simulink model "QUAD_EULER_MPC_FTSMC3"  (R2024b)
settings: Solver=ode1  StartTime=0.0  StopTime=30  FixedStep=0.001  RelTol=1e-3
values from neighbouring files (symbols this model uses):
  F1 = F1 + 2*(PSI_I'*C'*Q_z*C*PHI_I)    [Setup_MPC_SMC_Drone.m]
  F1_xy = F1_xy + 2*(PSI_xy_I'*C_xy'*Q_xy*C_xy*PHI_xy_I)    [Setup_MPC_SMC_Drone.m]
  F2 = F2 - 2*(PSI_I'*C'*Q_z*pi_n)    [Setup_MPC_SMC_Drone.m]
  F2_xy = F2_xy - 2*(PSI_xy_I'*C_xy'*Q_xy*pi_n)    [Setup_MPC_SMC_Drone.m]
  F3 = F3 - 2*(pi_nu'*Qt_z)    [Setup_MPC_SMC_Drone.m]
  F3_xy = F3_xy - 2*(pi_nu'*R_xy)    [Setup_MPC_SMC_Drone.m]
  F4 = F4 + 2*(PSI_I'*C'*Qt_z*C*SumG)    [Setup_MPC_SMC_Drone.m]
  g = 9.81    [Setup_MPC_SMC_Drone.m]
  G = [0;-g]    [Setup_MPC_SMC_Drone.m]
  H = H + 2*(PSI_I'*C'*Q_z*C*PSI_I + pi_nu'*Qt_z*pi_nu)    [Setup_MPC_SMC_Drone.m]
  H_xy = H_xy + 2*(PSI_xy_I'*C_xy'*Q_xy*C_xy*PSI_xy_I + pi_nu'*R_xy*pi_nu)    [Setup_MPC_SMC_Drone.m]
  J = diag([Jxx Jyy Jzz])    [Setup_MPC_SMC_Drone.m]
  m = 1.121    [Setup_MPC_SMC_Drone.m]
  N = 10    [Setup_MPC_SMC_Drone.m]
  N_xy = 10    [Setup_MPC_SMC_Drone.m]
  ny = size(C,1)    [Setup_MPC_SMC_Drone.m]
  ny_xy = size(C_xy,1)    [Setup_MPC_SMC_Drone.m]
  u_des = 0    [Setup_MPC_SMC_Drone.m]
  u_des_xy = [0;0]    [Setup_MPC_SMC_Drone.m]
undefined symbols (not defined in the file or in its folder): A_l, B_l, C_l, N_l, nr_l, nu, nu_l, phi_l, psi_l, Qu_l, Qy_l, ud_l
libraries: matrix_library x2, aerolibutil x2
settings Model: Creator=Jorge  LastModifiedBy=dr.gerardocastanon

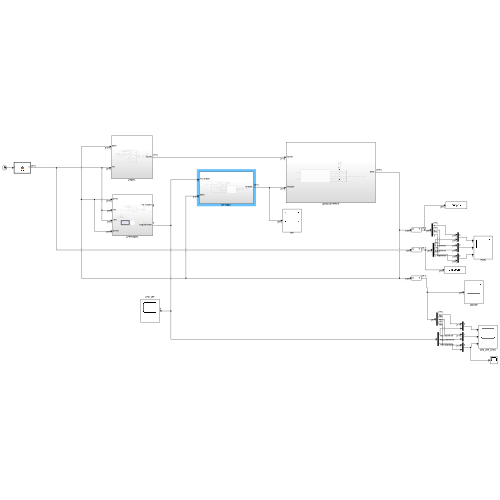
[thumbnail: Simulink's stored preview of the top-level diagram]
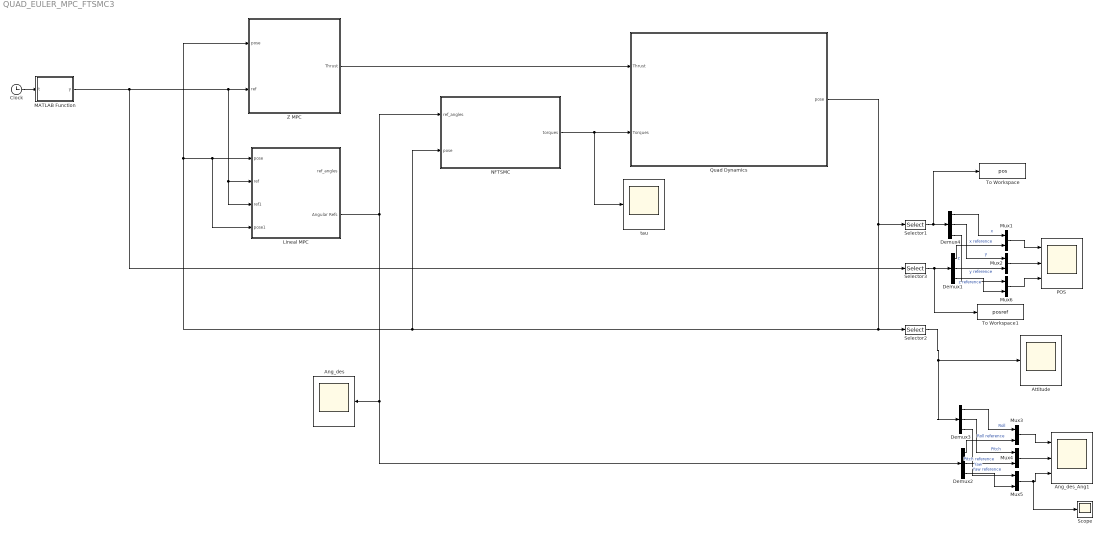
== system QUAD_EULER_MPC_FTSMC3 ==
  Ang_des : Scope
  Ang_des_Ang1 : Scope  NumInputPorts=3
  Attitude : Scope
  Clock : Clock
  Demux{1..4} (4 alike) : Demux  Outputs=3
  Lineal MPC : Subsystem
  MATLAB Function : MATLAB Function  TreatAsAtomicUnit=on
  Mux{1..6} (6 alike) : Mux  Inputs=2
  NFTSMC : Subsystem
  POS : Scope  NumInputPorts=3
  Quad Dynamics : Subsystem
  Scope : Scope
  Selector1 : Selector  InputPortWidth=15  IndexOptions=Starting index (dialog)  Indices=[1]  OutputSizes=3
  Selector2 : Selector  InputPortWidth=15  IndexOptions=Starting index (dialog)  Indices=[10]  OutputSizes=3
  Selector3 : Selector  InputPortWidth=4  IndexOptions=Starting index (dialog)  Indices=[1]  OutputSizes=3
  To Workspace : ToWorkspace  VariableName=pos  SampleTime=-1
  To Workspace1 : ToWorkspace  VariableName=posref  SampleTime=-1
  Z MPC : Subsystem
  tau : Scope
  wires:
  Quad Dynamics/1(pose) -> Selector1/1, Selector2/1, NFTSMC/2(pose), Z MPC/1(pose), Lineal MPC/4(pose1), Lineal MPC/1(pose)
  Z MPC/1(Thrust) -> Quad Dynamics/1(Thrust)
  MATLAB Function/1(y) -> Z MPC/2(ref), Lineal MPC/3(ref1), Lineal MPC/2(ref), Selector3/1
  Clock/1 -> MATLAB Function/1(t)
  Mux4/1 -> Ang_des_Ang1/2
  Mux5/1 -> Scope/1, Ang_des_Ang1/3
  Mux3/1 -> Ang_des_Ang1/1
  Mux2/1 -> POS/2
  Mux6/1 -> POS/3
  Mux1/1 -> POS/1
  Selector1/1 -> To Workspace/1, Demux4/1
  Selector3/1 -> To Workspace1/1, Demux1/1
  Demux3/1 -> Mux3/1  "Roll"
  Demux3/2 -> Mux4/1  "Pitch"
  Demux2/1 -> Mux3/2  "Roll reference"
  Demux3/3 -> Mux5/1  "Yaw"
  Demux2/2 -> Mux4/2  "Pitch reference"
  Demux2/3 -> Mux5/2  "Yaw reference"
  Demux4/1 -> Mux1/1  "x"
  Demux4/2 -> Mux2/1  "y"
  Demux1/1 -> Mux1/2  "x reference"
  Demux4/3 -> Mux6/1  "z"
  Demux1/2 -> Mux2/2  "y reference"
  Demux1/3 -> Mux6/2  "z reference"
  NFTSMC/1(torques) -> tau/1, Quad Dynamics/2(Torques)
  Selector2/1 -> Demux3/1, Attitude/1
  Lineal MPC/2(Angular Refs) -> Demux2/1, Ang_des/1, NFTSMC/1(ref_angles)

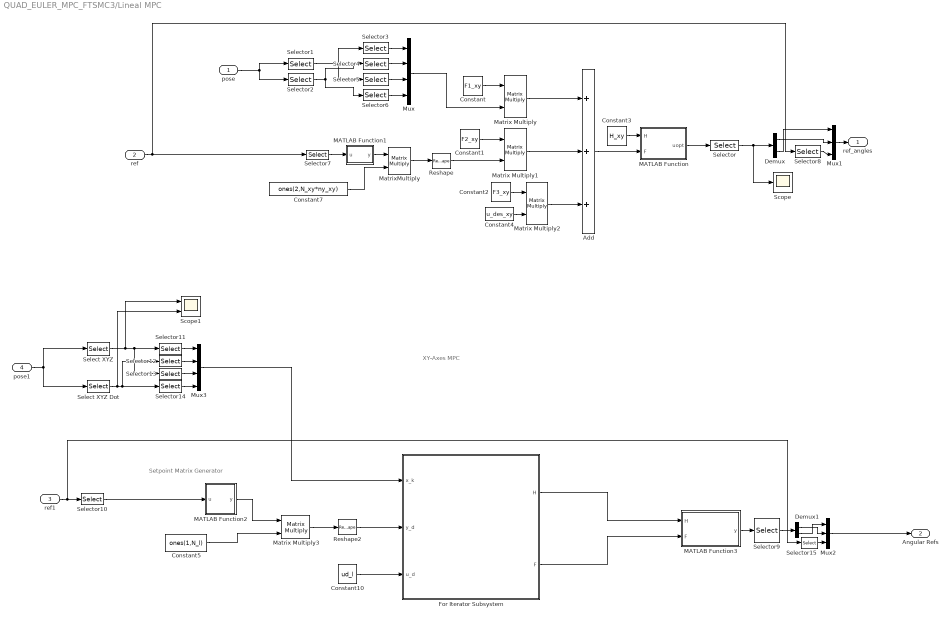
== system QUAD_EULER_MPC_FTSMC3/Lineal MPC ==
  note: Setpoint Matrix Generator
  note: XY-Axes MPC
  pose : Inport
  ref : Inport  Port=2
  ref1 : Inport  Port=3
  pose1 : Inport  Port=4
  Add : Sum  Inputs=+++
  Constant : Constant  Value=F1_xy
  Constant1 : Constant  Value=F2_xy
  Constant10 : Constant  Value=ud_l  VectorParams1D=off
  Constant2 : Constant  Value=F3_xy
  Constant3 : Constant  Value=H_xy
  Constant4 : Constant  Value=u_des_xy
  Constant5 : Constant  Value=ones(1,N_l)  VectorParams1D=off
  Constant7 : Constant  Value=ones(2,N_xy*ny_xy)
  Demux : Demux  Outputs=2
  Demux1 : Demux  Outputs=2
  For Iterator Subsystem : Subsystem  TreatAsAtomicUnit=on
  MATLAB Function : MATLAB Function  TreatAsAtomicUnit=on
  MATLAB Function1 : MATLAB Function  TreatAsAtomicUnit=on
  MATLAB Function2 : MATLAB Function  TreatAsAtomicUnit=on
  MATLAB Function3 : MATLAB Function  TreatAsAtomicUnit=on
  Matrix Multiply{,1..3} (4 alike) : Product  Multiplication=Matrix(*)
  MatrixMultiply : Product  Multiplication=Matrix(*)
  Mux : Mux
  Mux1 : Mux  Inputs=3
  Mux2 : Mux  Inputs=3
  Mux3 : Mux
  Reshape : Reshape  OutputDimensionality=Customize  OutputDimensions=[N_xy*ny_xy,1]
  Reshape2 : Reshape  OutputDimensionality=Customize  OutputDimensions=[N_l*nr_l,1]
  Scope : Scope
  Scope1 : Scope  NumInputPorts=2
  Select XYZ : Selector  InputPortWidth=15  IndexOptions=Index vector (dialog)  Indices=[1:3]  OutputSizes=1
  Select XYZ Dot : Selector  InputPortWidth=15  IndexOptions=Index vector (dialog)  Indices=[4:6]  OutputSizes=1
  Selector : Selector  InputPortWidth=20  IndexOptions=Starting index (dialog)  Indices=1  OutputSizes=2
  Selector1 : Selector  InputPortWidth=15  IndexOptions=Index vector (dialog)  Indices=[1 2]  OutputSizes=1
  Selector10 : Selector  InputPortWidth=4  IndexOptions=Index vector (dialog)  Indices=[1:2]  OutputSizes=1
  Selector11 : Selector  InputPortWidth=3  IndexOptions=Index vector (dialog)  Indices=[1]  OutputSizes=1
  Selector12 : Selector  InputPortWidth=3  IndexOptions=Index vector (dialog)  Indices=[1]  OutputSizes=1
  Selector13 : Selector  InputPortWidth=3  IndexOptions=Index vector (dialog)  Indices=[2]  OutputSizes=1
  Selector14 : Selector  InputPortWidth=3  IndexOptions=Index vector (dialog)  Indices=[2]  OutputSizes=1
  Selector15 : Selector  InputPortWidth=4  IndexOptions=Index vector (dialog)  Indices=4  OutputSizes=1
  Selector2 : Selector  InputPortWidth=15  IndexOptions=Index vector (dialog)  Indices=[4 5]  OutputSizes=1
  Selector3 : Selector  InputPortWidth=2  IndexOptions=Index vector (dialog)  Indices=1  OutputSizes=1
  Selector4 : Selector  InputPortWidth=2  IndexOptions=Index vector (dialog)  Indices=1  OutputSizes=1
  Selector5 : Selector  InputPortWidth=2  IndexOptions=Index vector (dialog)  Indices=2  OutputSizes=1
  Selector6 : Selector  InputPortWidth=2  IndexOptions=Index vector (dialog)  Indices=1  OutputSizes=1
  Selector7 : Selector  InputPortWidth=4  IndexOptions=Index vector (dialog)  Indices=[1:2]  OutputSizes=1
  Selector8 : Selector  InputPortWidth=4  IndexOptions=Index vector (dialog)  Indices=4  OutputSizes=1
  Selector9 : Selector  InputPortWidth=N_l*nu_l  IndexOptions=Index vector (dialog)  Indices=[1:2]  OutputSizes=1
  ref_angles : Outport
  Angular Refs : Outport  Port=2
  wires:
  Constant3/1 -> MATLAB Function/1(H)
  Add/1 -> MATLAB Function/2(F)
  MATLAB Function/1(uopt) -> Selector/1
  Selector/1 -> Demux/1, Scope/1
  pose/1 -> Selector2/1, Selector1/1
  Selector1/1 -> Selector3/1, Selector5/1
  Selector2/1 -> Selector4/1, Selector6/1
  Selector3/1 -> Mux/1
  Selector4/1 -> Mux/2
  Selector5/1 -> Mux/3
  Selector6/1 -> Mux/4
  Constant/1 -> Matrix Multiply/1
  Mux/1 -> Matrix Multiply/2
  Matrix Multiply/1 -> Add/1
  Matrix Multiply1/1 -> Add/2
  Constant1/1 -> Matrix Multiply1/1
  Constant7/1 -> MatrixMultiply/2
  ref/1 -> Selector8/1, Selector7/1
  MatrixMultiply/1 -> Reshape/1
  Reshape/1 -> Matrix Multiply1/2
  Matrix Multiply2/1 -> Add/3
  Constant2/1 -> Matrix Multiply2/1
  Constant4/1 -> Matrix Multiply2/2
  Selector7/1 -> MATLAB Function1/1(u)
  MATLAB Function1/1(y) -> MatrixMultiply/1
  Mux1/1 -> ref_angles/1
  Demux/2 -> Mux1/1
  Demux/1 -> Mux1/2
  Selector8/1 -> Mux1/3
  Constant10/1 -> For Iterator Subsystem/3(u_d)
  Selector13/1 -> Mux3/3
  Selector10/1 -> MATLAB Function2/1(u)
  Selector9/1 -> Demux1/1
  Select XYZ/1 -> Scope1/1, Selector13/1, Selector11/1
  Demux1/1 -> Mux2/2
  For Iterator Subsystem/1(H) -> MATLAB Function3/1(H)
  Selector14/1 -> Mux3/4
  MATLAB Function2/1(y) -> Matrix Multiply3/1
  Constant5/1 -> Matrix Multiply3/2
  Selector15/1 -> Mux2/3
  Selector12/1 -> Mux3/2
  MATLAB Function3/1(y) -> Selector9/1
  Selector11/1 -> Mux3/1
  Matrix Multiply3/1 -> Reshape2/1
  ref1/1 -> Selector15/1, Selector10/1
  Select XYZ Dot/1 -> Scope1/2, Selector12/1, Selector14/1
  Mux3/1 -> For Iterator Subsystem/1(x_k)
  Reshape2/1 -> For Iterator Subsystem/2(y_d)
  For Iterator Subsystem/2(F) -> MATLAB Function3/2(F)
  pose1/1 -> Select XYZ Dot/1, Select XYZ/1
  Demux1/2 -> Mux2/1
  Mux2/1 -> Angular Refs/1

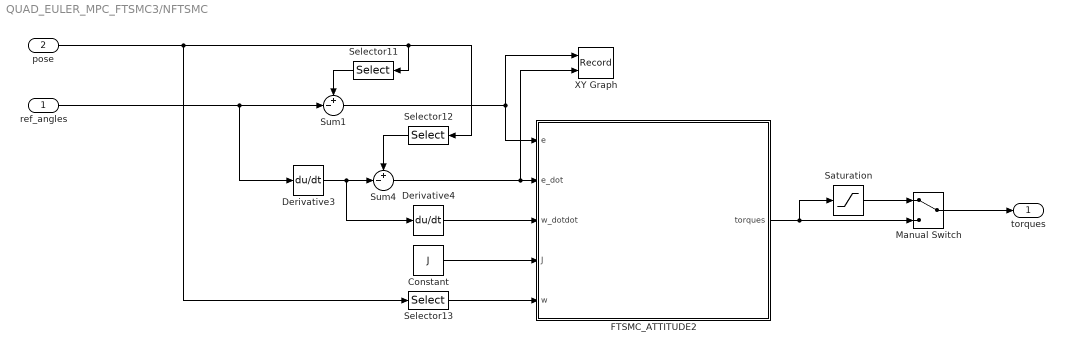
== system QUAD_EULER_MPC_FTSMC3/NFTSMC ==
  ref_angles : Inport
  pose : Inport  Port=2
  Constant : Constant  Value=J
  Derivative3 : Derivative
  Derivative4 : Derivative
  FTSMC_ATTITUDE2 : Subsystem
  Manual Switch : ManualSwitch
  Saturation : Saturate  UpperLimit=1  LowerLimit=-1
  Selector11 : Selector  InputPortWidth=15  IndexOptions=Starting index (dialog)  Indices=[10]  OutputSizes=3
  Selector12 : Selector  InputPortWidth=15  IndexOptions=Starting index (dialog)  Indices=[13]  OutputSizes=3
  Selector13 : Selector  InputPortWidth=15  IndexOptions=Starting index (dialog)  Indices=[13]  OutputSizes=3
  Sum1 : Sum  Inputs=+-|
  Sum4 : Sum  Inputs=+-|
  XY Graph : Record  FileSettingsInternal="{\"entries\":[{\"content\":{\"excelSettings\":{\"content\":{},\"type\":\"Streamout.ExcelSettings\"}},\"type\":\"Streamout.FileSettingStorage\",\"uuid\":\"\"}],\"packageUris\":[\"http:\\/\\/schema.mathworks.com\\/mf0\\/streamout_blocks\\/R2020a\"],\"version\":\"1.0\"}"  Layout=[1 1]  SignalsInternal="{\"entries\":[{\"content\":{\"signals\":[{\"content\":{\"blockPath\":[],\"dimensions\":[3,1],\"domain\":\"\",\"hasChildren\":true,\"lineColor\":\"#77ac30\",\"lineWidth\":2,\"port\":1,\"sid\":[\"\"],\"signalID\":1,\"signalName\":\"Sum1\"},\"type\":\"RecordBlkView.Signal\",\"uuid\":\"\"},{\"content\":{\"blockPath\":[],\"channel\":[1,1],\"dimensions\":[3,1],\"domain\":\"\",\"lineColor\":\"#ff13a6\",\"lineWidth\":2,\"parentID\":1,\"plots\":[ 1 ],\"port\":1,\"sid\":[\"\"],\"signalID\":2,\"signalName\":\"Sum1\"},\"type\":\"RecordBlkView.Signal\",\"uuid\":\"\"},{\"content\":{\"blockPath\":[],\"dimensions\":[3,1],\"domain\":\"\",\"hasChildren\":true,\"lineColor\":\"#a2142f\",\"lineWidth\":2,\"port\":2,\"sid\":[\"\"],\"signalID\":3,\"signalName\":\"Sum4\"},\"type\":\"RecordBlkView.Signal\",\"uuid\":\"\"},{\"content\":{\"blockPath\":[],\"channel\":[1,1],\"dimensions\":[3,1],\"domain\":\"\",\"lineColor\":\"#22b573\",\"lineWidth\":2,\"parentID\":3,\"plots\":[ 1 ],\"port\":2,\"sid\":[\"\"],\"signalID\":4,\"signalName\":\"Sum4\"},\"type\":\"RecordBlkView.Signal\",\"uuid\":\"\"},{\"content\":{\"blockPath\":[],\"channel\":[2,1],\"dimensions\":[3,1],\"domain\":\"\",\"lineColor\":\"#0072bd\",\"lineWidth\":2,\"parentID\":1,\"port\":1,\"sid\":[\"\"],\"signalID\":5,\"signalName\":\"Sum1\"},\"type\":\"RecordBlkView.Signal\",\"uuid\":\"\"},{\"content\":{\"blockPath\":[],\"channel\":[3,1],\"dimensions\":[3,1],\"domain\":\"\",\"lineColor\":\"#d95319\",\"lineWidth\":2,\"parentID\":1,\"port\":1,\"sid\":[\"\"],\"signalID\":6,\"signalName\":\"Sum1\"},\"type\":\"RecordBlkView.Signal\",\"uuid\":\"\"},{\"content\":{\"blockPath\":[],\"channel\":[2,1],\"dimensions\":[3,1],\"domain\":\"\",\"lineColor\":\"#edb120\",\"lineWidth\":2,\"parentID\":3,\"port\":2,\"sid\":[\"\"],\"signalID\":7,\"signalName\":\"Sum4\"},\"type\":\"RecordBlkView.Signal\",\"uuid\":\"\"},{\"content\":{\"blockPath\":[],\"channel\":[3,1],\"dimensions\":[3,1],\"domain\":\"\",\"lineColor\":\"#7e2f8e\",\"lineWidth\":2,\"parentID\":3,\"port\":2,\"sid\":[\"\"],\"signalID\":8,\"signalName\":\"Sum4\"},\"type\":\"RecordBlkView.Signal\",\"uuid\":\"\"}]},\"type\":\"RecordBlkView.InputSignals\",\"uuid\":\"\"}],\"packageUris\":[\"http:\\/\\/schema.mathworks.com\\/mf0\\/streamout_blocks\\/R2020a\"],\"version\":\"1.0\"}"  VisualizationBindings="{\"xyplotplugin\":{\"info\":[{\"series\":[{\"bindingParametersList\":[{\"parameter\":\"X-Axis\",\"signalID\":2,\"signalName\":\"Sum1(1,1)\"},{\"parameter\":\"Y-Axis\",\"signalID\":4,\"signalName\":\"Sum4(1,1)\"}],\"seriesID\":0}],\"subplotID\":1}]}}"  CompatibilityTag=XY
  torques : Outport
  wires:
  Sum4/1 -> XY Graph/2, FTSMC_ATTITUDE2/2(e_dot)
  Sum1/1 -> XY Graph/1, FTSMC_ATTITUDE2/1(e)
  Selector11/1 -> Sum1/1
  ref_angles/1 -> Sum1/2, Derivative3/1
  Selector13/1 -> FTSMC_ATTITUDE2/5(w)
  Selector12/1 -> Sum4/1
  Derivative3/1 -> Sum4/2, Derivative4/1
  Derivative4/1 -> FTSMC_ATTITUDE2/3(w_dotdot)
  pose/1 -> Selector13/1, Selector11/1, Selector12/1
  Constant/1 -> FTSMC_ATTITUDE2/4(J)
  FTSMC_ATTITUDE2/1(torques) -> Saturation/1, Manual Switch/2
  Saturation/1 -> Manual Switch/1
  Manual Switch/1 -> torques/1

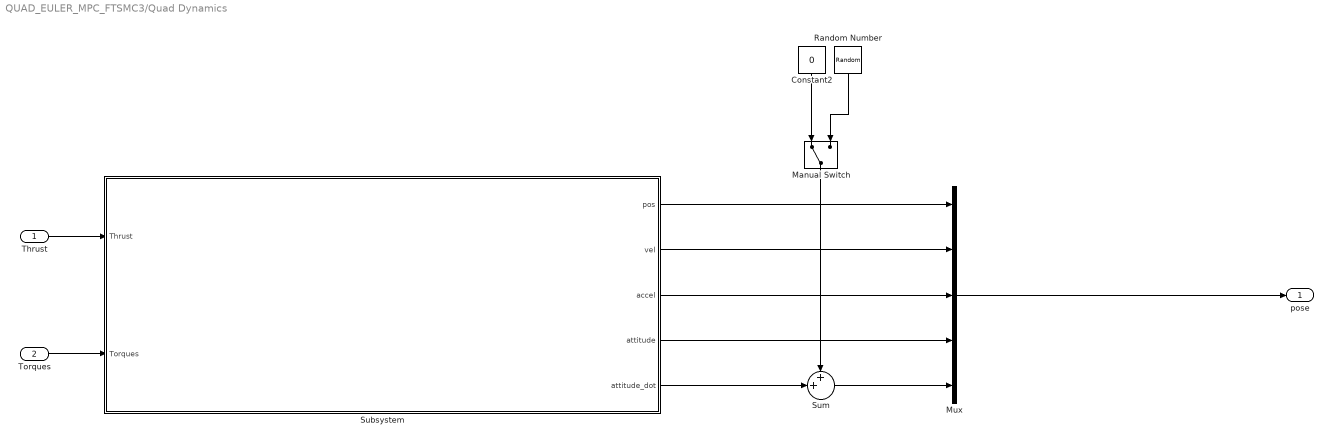
== system QUAD_EULER_MPC_FTSMC3/Quad Dynamics ==
  Thrust : Inport
  Torques : Inport  Port=2
  Constant2 : Constant  Value=0
  Manual Switch : ManualSwitch
  Mux : Mux  Inputs=5
  Random Number : RandomNumber  Variance=0.01  SampleTime=0.1
  Subsystem : Subsystem
  Sum : Sum  Inputs=++|
  pose : Outport
  wires:
  Subsystem/1(pos) -> Mux/1
  Subsystem/2(vel) -> Mux/2
  Subsystem/3(accel) -> Mux/3
  Subsystem/4(attitude) -> Mux/4
  Thrust/1 -> Subsystem/1(Thrust)
  Torques/1 -> Subsystem/2(Torques)
  Mux/1 -> pose/1
  Manual Switch/1 -> Sum/1
  Random Number/1 -> Manual Switch/2
  Subsystem/5(attitude_dot) -> Sum/2
  Constant2/1 -> Manual Switch/1
  Sum/1 -> Mux/5

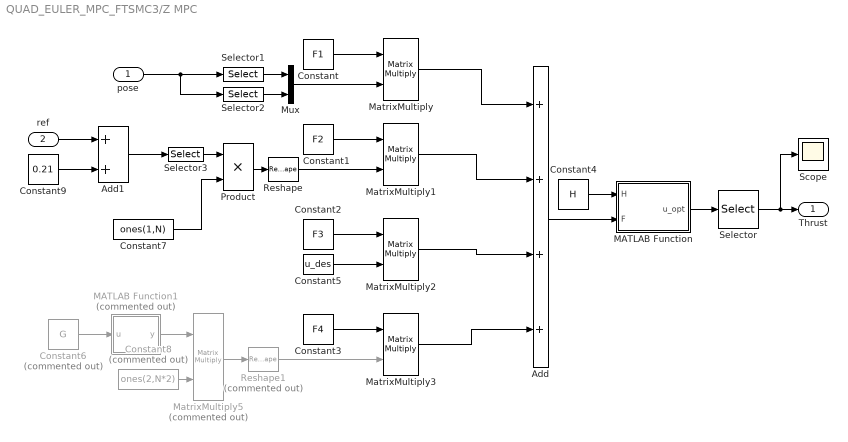
== system QUAD_EULER_MPC_FTSMC3/Z MPC ==
  pose : Inport
  ref : Inport  Port=2
  Add : Sum  Inputs=++++
  Add1 : Sum
  Constant : Constant  Value=F1
  Constant1 : Constant  Value=F2
  Constant2 : Constant  Value=F3
  Constant3 : Constant  Value=F4
  Constant4 : Constant  Value=H
  Constant5 : Constant  Value=u_des
  Constant6 : Constant  Commented=on  Value=G
  Constant7 : Constant  Value=ones(1,N)
  Constant8 : Constant  Commented=on  Value=ones(2,N*2)
  Constant9 : Constant  Value=0.21
  MATLAB Function : MATLAB Function  TreatAsAtomicUnit=on
  MATLAB Function1 : MATLAB Function  Commented=on  TreatAsAtomicUnit=on
  MatrixMultiply{,1..3} (4 alike) : Product  Multiplication=Matrix(*)
  MatrixMultiply5 : Product  Commented=on  Multiplication=Matrix(*)
  Mux : Mux  Inputs=2
  Product : Product
  Reshape : Reshape  OutputDimensionality=Customize  OutputDimensions=[N*ny,1]
  Reshape1 : Reshape  Commented=on  OutputDimensionality=Customize  OutputDimensions=[2*N,1]
  Scope : Scope
  Selector : Selector  InputPortWidth=N*nu  IndexOptions=Index vector (dialog)  Indices=1  OutputSizes=1
  Selector1 : Selector  InputPortWidth=15  IndexOptions=Index vector (dialog)  Indices=3  OutputSizes=1
  Selector2 : Selector  InputPortWidth=15  IndexOptions=Index vector (dialog)  Indices=6  OutputSizes=1
  Selector3 : Selector  InputPortWidth=4  IndexOptions=Index vector (dialog)  Indices=3  OutputSizes=1
  Thrust : Outport
  wires:
  Add/1 -> MATLAB Function/2(F)
  Constant4/1 -> MATLAB Function/1(H)
  MATLAB Function/1(u_opt) -> Selector/1
  Selector/1 -> Scope/1, Thrust/1
  Constant/1 -> MatrixMultiply/1
  MatrixMultiply/1 -> Add/1
  MatrixMultiply1/1 -> Add/2
  MatrixMultiply2/1 -> Add/3
  MatrixMultiply3/1 -> Add/4
  Mux/1 -> MatrixMultiply/2
  Selector2/1 -> Mux/2
  Selector1/1 -> Mux/1
  pose/1 -> Selector2/1, Selector1/1
  Constant1/1 -> MatrixMultiply1/1
  Constant5/1 -> MatrixMultiply2/2
  Constant2/1 -> MatrixMultiply2/1
  Constant7/1 -> Product/2
  Selector3/1 -> Product/1
  Product/1 -> Reshape/1
  Reshape/1 -> MatrixMultiply1/2
  Constant8/1 -> MatrixMultiply5/2
  Constant6/1 -> MATLAB Function1/1(u)
  MatrixMultiply5/1 -> Reshape1/1
  Reshape1/1 -> MatrixMultiply3/2
  Constant3/1 -> MatrixMultiply3/1
  MATLAB Function1/1(y) -> MatrixMultiply5/1
  Add1/1 -> Selector3/1
  ref/1 -> Add1/1
  Constant9/1 -> Add1/2

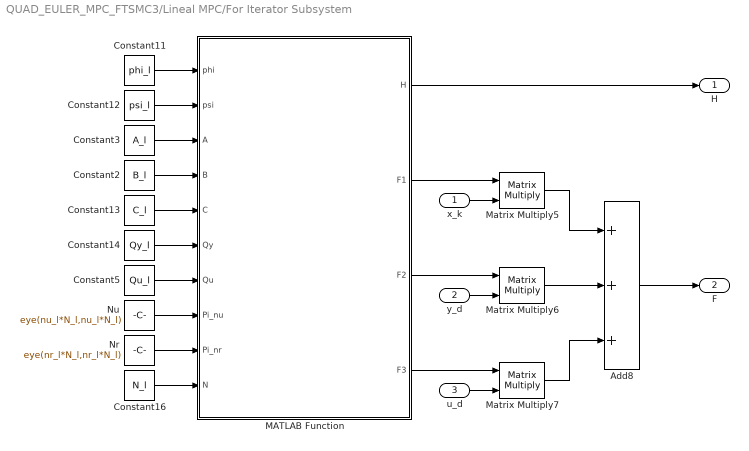
== system QUAD_EULER_MPC_FTSMC3/Lineal MPC/For Iterator Subsystem ==
  x_k : Inport
  y_d : Inport  Port=2
  u_d : Inport  Port=3
  Add8 : Sum  Inputs=+++
  Constant11 : Constant  Value=phi_l
  Constant12 : Constant  Value=psi_l
  Constant13 : Constant  Value=C_l
  Constant14 : Constant  Value=Qy_l
  Constant16 : Constant  Value=N_l
  Constant2 : Constant  Value=B_l
  Constant3 : Constant  Value=A_l
  Constant5 : Constant  Value=Qu_l
  MATLAB Function : MATLAB Function  TreatAsAtomicUnit=on
  Matrix Multiply5 : Product  Multiplication=Matrix(*)
  Matrix Multiply6 : Product  Multiplication=Matrix(*)
  Matrix Multiply7 : Product  Multiplication=Matrix(*)
  Nr : Constant  Value=eye(nr_l*N_l,nr_l*N_l)
  Nu : Constant  Value=eye(nu_l*N_l,nu_l*N_l)
  H : Outport
  F : Outport  Port=2
  wires:
  x_k/1 -> Matrix Multiply5/2
  y_d/1 -> Matrix Multiply6/2
  u_d/1 -> Matrix Multiply7/2
  Matrix Multiply6/1 -> Add8/2
  Matrix Multiply5/1 -> Add8/1
  Matrix Multiply7/1 -> Add8/3
  Add8/1 -> F/1
  Nr/1 -> MATLAB Function/9(Pi_nr)
  Nu/1 -> MATLAB Function/8(Pi_nu)
  Constant16/1 -> MATLAB Function/10(N)
  Constant11/1 -> MATLAB Function/1(phi)
  Constant14/1 -> MATLAB Function/6(Qy)
  Constant12/1 -> MATLAB Function/2(psi)
  Constant13/1 -> MATLAB Function/5(C)
  Constant2/1 -> MATLAB Function/4(B)
  Constant3/1 -> MATLAB Function/3(A)
  MATLAB Function/4(F3) -> Matrix Multiply7/1
  MATLAB Function/3(F2) -> Matrix Multiply6/1
  MATLAB Function/2(F1) -> Matrix Multiply5/1
  MATLAB Function/1(H) -> H/1
  Constant5/1 -> MATLAB Function/7(Qu)

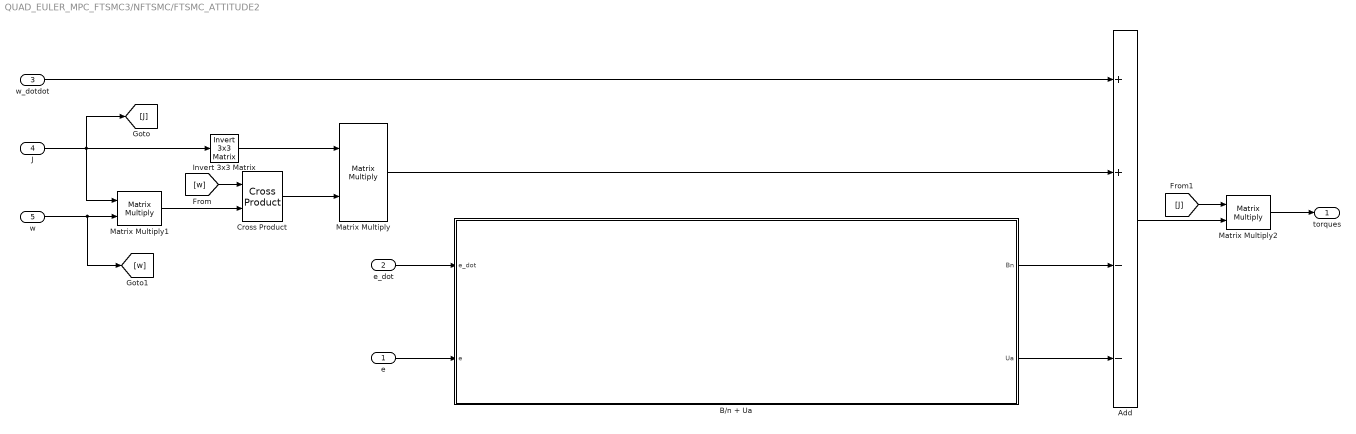
== system QUAD_EULER_MPC_FTSMC3/NFTSMC/FTSMC_ATTITUDE2 ==
  e : Inport
  e_dot : Inport  Port=2
  w_dotdot : Inport  Port=3
  J : Inport  Port=4
  w : Inport  Port=5
  Add : Sum  Inputs=++--
  B/n + Ua : Subsystem
  Cross Product : matrix_library/Cross Product
  Invert 3x3 Matrix : aerolibutil/Invert  3x3 Matrix
  Matrix Multiply : Product  Multiplication=Matrix(*)
  Matrix Multiply1 : Product  Multiplication=Matrix(*)
  Matrix Multiply2 : Product  Multiplication=Matrix(*)
  torques : Outport
  wires:
  J/1 -> [J], Matrix Multiply1/1, Invert 3x3 Matrix/1
  Invert 3x3 Matrix/1 -> Matrix Multiply/1
  Cross Product/1 -> Matrix Multiply/2
  Matrix Multiply1/1 -> Cross Product/2
  w/1 -> [w], Matrix Multiply1/2
  [w] -> Cross Product/1
  w_dotdot/1 -> Add/1
  Matrix Multiply/1 -> Add/2
  Add/1 -> Matrix Multiply2/2
  Matrix Multiply2/1 -> torques/1
  [J] -> Matrix Multiply2/1
  B/n + Ua/1(Bn) -> Add/3
  B/n + Ua/2(Ua) -> Add/4
  e_dot/1 -> B/n + Ua/1(e_dot)
  e/1 -> B/n + Ua/2(e)

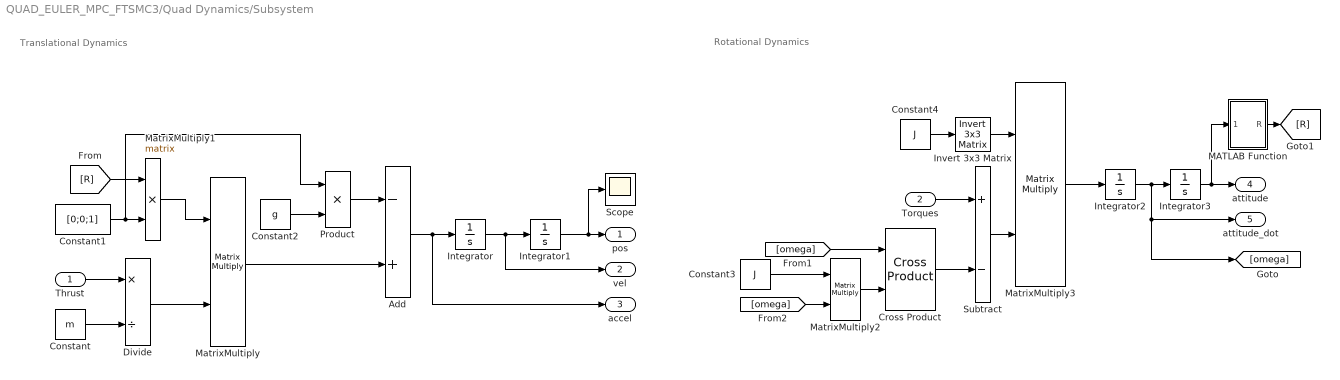
== system QUAD_EULER_MPC_FTSMC3/Quad Dynamics/Subsystem ==
  note: Rotational Dynamics
  note: Translational Dynamics
  Thrust : Inport
  Torques : Inport  Port=2
  Add : Sum  Inputs=-+
  Constant : Constant  Value=m
  Constant1 : Constant  Value=[0;0;1]
  Constant2 : Constant  Value=g
  Constant3 : Constant  Value=J
  Constant4 : Constant  Value=J
  Cross Product : matrix_library/Cross Product
  Divide : Product  Inputs=*/
  Integrator{,1..3} (4 alike) : Integrator
  Invert 3x3 Matrix : aerolibutil/Invert  3x3 Matrix
  MATLAB Function : MATLAB Function  TreatAsAtomicUnit=on
  MatrixMultiply{,1..3} (4 alike) : Product  Multiplication=Matrix(*)
  Product : Product
  Scope : Scope
  Subtract : Sum  Inputs=+-
  pos : Outport
  vel : Outport  Port=2
  accel : Outport  Port=3
  attitude : Outport  Port=4
  attitude_dot : Outport  Port=5
  wires:
  Constant/1 -> Divide/2
  MatrixMultiply1/1 -> MatrixMultiply/1
  Integrator2/1 -> [omega], attitude_dot/1, Integrator3/1
  Constant2/1 -> Product/2
  Integrator1/1 -> Scope/1, pos/1
  Integrator/1 -> vel/1, Integrator1/1
  Constant4/1 -> Invert 3x3 Matrix/1
  [omega] -> Cross Product/1
  Constant3/1 -> MatrixMultiply2/1
  [omega] -> MatrixMultiply2/2
  Cross Product/1 -> Subtract/2
  Divide/1 -> MatrixMultiply/2
  Torques/1 -> Subtract/1
  [R] -> MatrixMultiply1/1
  MatrixMultiply/1 -> Add/2
  Integrator3/1 -> MATLAB Function/1(att), attitude/1
  MATLAB Function/1(R) -> [R]
  Constant1/1 -> Product/1, MatrixMultiply1/2
  MatrixMultiply3/1 -> Integrator2/1
  Add/1 -> accel/1, Integrator/1
  MatrixMultiply2/1 -> Cross Product/2
  Subtract/1 -> MatrixMultiply3/2
  Thrust/1 -> Divide/1
  Product/1 -> Add/1
  Invert 3x3 Matrix/1 -> MatrixMultiply3/1

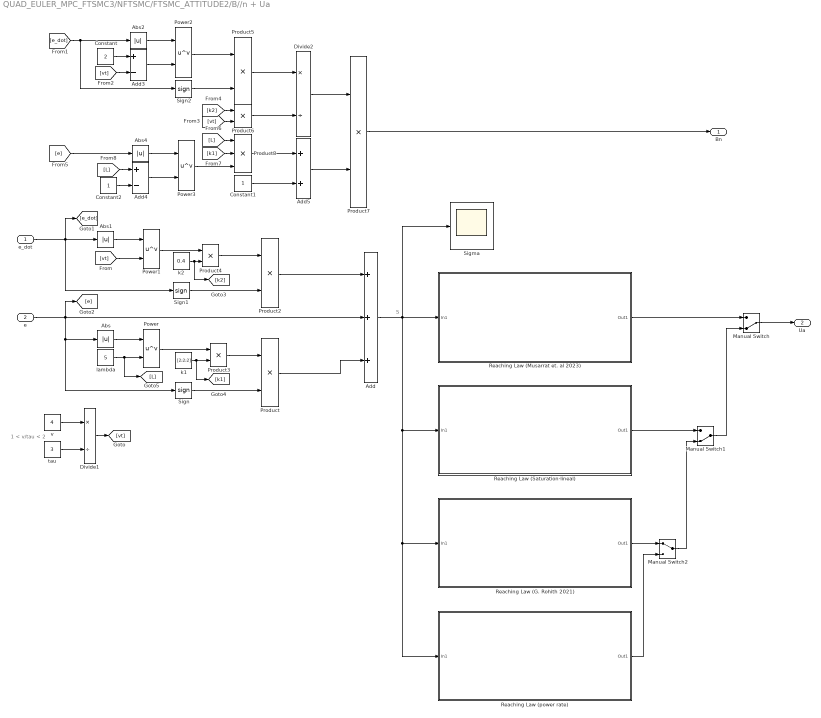
== system QUAD_EULER_MPC_FTSMC3/NFTSMC/FTSMC_ATTITUDE2/B//n + Ua ==
  note: S
  note: 1 < v/tau < 2
  e_dot : Inport
  e : Inport  Port=2
  Abs{,1..2,4} (4 alike) : Abs  SaturateOnIntegerOverflow=off
  Add : Sum  Inputs=+++
  Add3 : Sum  Inputs=+-
  Add4 : Sum  Inputs=+-
  Add5 : Sum
  Constant : Constant  Value=2
  Constant1 : Constant
  Constant2 : Constant
  Divide1 : Product  Inputs=*/
  Divide2 : Product  Inputs=*/
  Manual Switch : ManualSwitch  CurrentSetting=0
  Manual Switch1 : ManualSwitch  CurrentSetting=0
  Manual Switch2 : ManualSwitch
  Power{,1..3} (4 alike) : Math  Operator=pow
  Product{,2..7} (7 alike) : Product
  Product8 : Product  Inputs=3
  Reaching Law (G. Rohith 2021) : Subsystem
  Reaching Law (Musarrat et. al 2023) : Subsystem
  Reaching Law (Saturation-lineal) : Subsystem
  Reaching Law (power rate) : Subsystem
  Sigma : Scope
  Sign : Signum
  Sign1 : Signum
  Sign2 : Signum
  k1 : Constant  Value=[2;2;2]
  k2 : Constant  Value=0.4
  lambda : Constant  Value=5
  tau : Constant  Value=3
  v : Constant  Value=4
  Bn : Outport
  Ua : Outport  Port=2
  wires:
  Constant1/1 -> Add5/2
  [k2] -> Product6/1
  Power3/1 -> Product8/3
  Product5/1 -> Divide2/1
  Product6/1 -> Divide2/2
  k1/1 -> Product3/2, [k1]
  tau/1 -> Divide1/2
  lambda/1 -> [L], Power/2
  [vt] -> Power1/2
  [vt] -> Product6/2
  [e_dot] -> Sign2/1, Abs2/1
  Power1/1 -> Product4/1
  Sign1/1 -> Product2/2
  Add4/1 -> Power3/2
  [k1] -> Product8/2
  Product/1 -> Add/3
  e/1 -> [e], Abs/1, Sign/1, Add/2
  Constant2/1 -> Add4/2
  v/1 -> Divide1/1
  Sign/1 -> Product/2
  k2/1 -> [k2], Product4/2
  Sign2/1 -> Product5/2
  Add3/1 -> Power2/2
  Power2/1 -> Product5/1
  Abs2/1 -> Power2/1
  Abs/1 -> Power/1
  Constant/1 -> Add3/1
  [vt] -> Add3/2
  [L] -> Add4/1
  Abs1/1 -> Power1/1
  [L] -> Product8/1
  e_dot/1 -> [e_dot], Abs1/1, Sign1/1
  Add5/1 -> Product7/2
  [e] -> Abs4/1
  Divide2/1 -> Product7/1
  Product3/1 -> Product/1
  Power/1 -> Product3/1
  Product8/1 -> Add5/1
  Product2/1 -> Add/1
  Abs4/1 -> Power3/1
  Product4/1 -> Product2/1
  Divide1/1 -> [vt]
  Product7/1 -> Bn/1
  Add/1 -> Sigma/1, Reaching Law (G. Rohith 2021)/1(In1), Reaching Law (power rate)/1(In1), Reaching Law (Saturation-lineal)/1(In1), Reaching Law (Musarrat et. al 2023)/1(In1)
  Reaching Law (Musarrat et. al 2023)/1(Out1) -> Manual Switch/1
  Manual Switch/1 -> Ua/1
  Reaching Law (Saturation-lineal)/1(Out1) -> Manual Switch1/1
  Manual Switch1/1 -> Manual Switch/2
  Reaching Law (G. Rohith 2021)/1(Out1) -> Manual Switch2/1
  Reaching Law (power rate)/1(Out1) -> Manual Switch2/2
  Manual Switch2/1 -> Manual Switch1/2

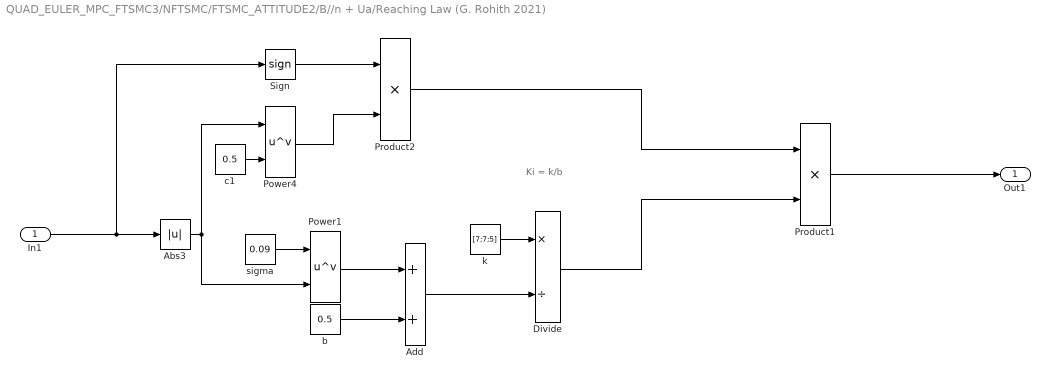
== system QUAD_EULER_MPC_FTSMC3/NFTSMC/FTSMC_ATTITUDE2/B//n + Ua/Reaching Law (G. Rohith 2021) ==
  note: Ki = k/b
  In1 : Inport
  Abs3 : Abs  SaturateOnIntegerOverflow=off
  Add : Sum
  Divide : Product  Inputs=*/
  Power1 : Math  Operator=pow
  Power4 : Math  Operator=pow
  Product1 : Product
  Product2 : Product
  Sign : Signum
  b : Constant  Value=0.5
  c1 : Constant  Value=0.5
  k : Constant  Value=[7;7;5]
  sigma : Constant  Value=0.09
  Out1 : Outport
  wires:
  Power4/1 -> Product2/2
  c1/1 -> Power4/2
  Sign/1 -> Product2/1
  Abs3/1 -> Power1/2, Power4/1
  In1/1 -> Sign/1, Abs3/1
  Product1/1 -> Out1/1
  Product2/1 -> Product1/1
  sigma/1 -> Power1/1
  Power1/1 -> Add/1
  k/1 -> Divide/1
  Add/1 -> Divide/2
  Divide/1 -> Product1/2
  b/1 -> Add/2

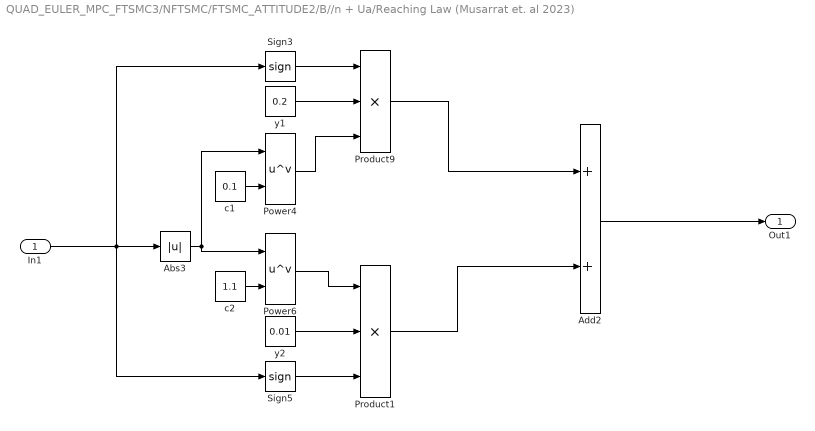
== system QUAD_EULER_MPC_FTSMC3/NFTSMC/FTSMC_ATTITUDE2/B//n + Ua/Reaching Law (Musarrat et. al 2023) ==
  In1 : Inport
  Abs3 : Abs  SaturateOnIntegerOverflow=off
  Add2 : Sum
  Power4 : Math  Operator=pow
  Power6 : Math  Operator=pow
  Product1 : Product  Inputs=3
  Product9 : Product  Inputs=3
  Sign3 : Signum
  Sign5 : Signum
  c1 : Constant  Value=0.1
  c2 : Constant  Value=1.1
  y1 : Constant  Value=0.2
  y2 : Constant  Value=0.01
  Out1 : Outport
  wires:
  Add2/1 -> Out1/1
  Product1/1 -> Add2/2
  y2/1 -> Product1/2
  c1/1 -> Power4/2
  Power4/1 -> Product9/3
  Abs3/1 -> Power4/1, Power6/1
  Sign5/1 -> Product1/3
  Sign3/1 -> Product9/1
  In1/1 -> Sign5/1, Sign3/1, Abs3/1
  Power6/1 -> Product1/1
  Product9/1 -> Add2/1
  c2/1 -> Power6/2
  y1/1 -> Product9/2

== system QUAD_EULER_MPC_FTSMC3/NFTSMC/FTSMC_ATTITUDE2/B//n + Ua/Reaching Law (Saturation-lineal) ==
  In1 : Inport
  Add2 : Sum
  Gain : Gain  Gain=0.01
  Product9 : Product
  Saturation : Saturate
  y1 : Constant  Value=10
  Out1 : Outport
  wires:
  Add2/1 -> Out1/1
  Saturation/1 -> Product9/1
  In1/1 -> Saturation/1, Gain/1
  Product9/1 -> Add2/1
  y1/1 -> Product9/2
  Gain/1 -> Add2/2

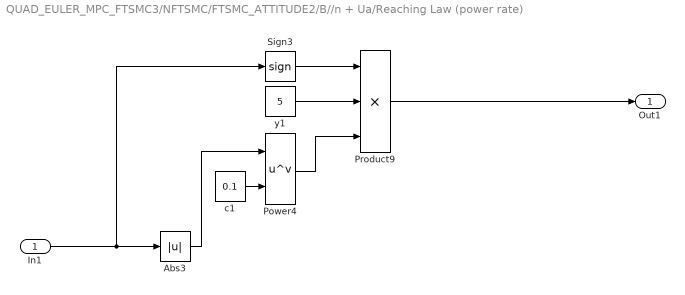
== system QUAD_EULER_MPC_FTSMC3/NFTSMC/FTSMC_ATTITUDE2/B//n + Ua/Reaching Law (power rate) ==
  In1 : Inport
  Abs3 : Abs  SaturateOnIntegerOverflow=off
  Power4 : Math  Operator=pow
  Product9 : Product  Inputs=3
  Sign3 : Signum
  c1 : Constant  Value=0.1
  y1 : Constant  Value=5
  Out1 : Outport
  wires:
  Product9/1 -> Out1/1
  c1/1 -> Power4/2
  Power4/1 -> Product9/3
  Abs3/1 -> Power4/1
  Sign3/1 -> Product9/1
  In1/1 -> Sign3/1, Abs3/1
  y1/1 -> Product9/2

== matlab function QUAD_EULER_MPC_FTSMC3/Z MPC/MATLAB Function ==
  data: H input; u_opt output; F input
function u_opt = fcn(H,F)

u_opt = -H\F;

== matlab function QUAD_EULER_MPC_FTSMC3/Lineal MPC/MATLAB Function ==
  data: H input; uopt output; F input
function uopt = fcn(H,F)

uopt = -H\F;

== matlab function QUAD_EULER_MPC_FTSMC3/Z MPC/MATLAB Function1 ==
  data: u input; y output
function y = fcn(u)

y = [u(1) u(2)];

== matlab function QUAD_EULER_MPC_FTSMC3/Quad Dynamics/Subsystem/MATLAB Function ==
  data: att input; R output
function R = fcn(att)
phi = att(1);
theta = att(2);
psi = att(3);

R = [
cos(psi)*cos(theta), cos(psi)*sin(theta)*sin(phi) - cos(phi)*sin(psi), cos(psi)*cos(phi)*sin(theta)+sin(phi)*sin(psi);
cos(theta)*sin(psi), sin(psi)*sin(phi)*sin(theta) + cos(phi)*cos(psi), sin(psi)*cos(phi)*sin(theta)-cos(psi)*sin(phi);
-sin(theta),cos(theta)*sin(phi), cos(phi)*cos(theta);
];

== matlab function QUAD_EULER_MPC_FTSMC3/Lineal MPC/MATLAB Function1 ==
  data: u input; y output
function y = fcn(u)

y = [u(1),u(2)];

== matlab function QUAD_EULER_MPC_FTSMC3/MATLAB Function ==
  data: t input; y output
function y = fcn(t)

% y = [sin(0.5*t);cos(0.5*t);0.1*t;0];

% y = [2*cos(1*t/10);sin(2*t/10);1;0];

% if t < 5*pi/2
%     y = [1;2;0;0];
% elseif t > 5*pi/2
%     y = [2*cos(t);2*sin(t);0;0];
% else
%     y = [0;0;0;0];
% end

if t < 8
    y = [0;1;0;0];
elseif t > 18
    y = [0;1;1;0];
else
    y = [0;0;0;0];
end

== matlab function QUAD_EULER_MPC_FTSMC3/Lineal MPC/For Iterator Subsystem/MATLAB Function ==
  data: phi input; H output; psi input; A input; B input; C input; Qy input; Qu input; Pi_nu input; Pi_nr input; N input; F1 output; F2 output; F3 output
function [H,F1,F2,F3] = fcn(phi,psi,A,B,C,Qy,Qu,Pi_nu,Pi_nr,N)

% Size variables definition
[n,nu] = size(B);
nr = size(C,1);

H = zeros(20,20);     % size = (N*nu,N*nu)
F1 = zeros(20,4);
F2 = zeros(20,20);
F3 = zeros(20,2);

for i = 1:N
    psi_i = psi((i*n)-(n-1):i*(n),:);
    phi_i = phi((i*n)-(n-1):i*(n),:);

    Pi_nu_i = Pi_nu((i*nu)-(nu-1):i*(nu),:);
    Pi_nr_i = Pi_nr((i*nu)-(nu-1):i*(nu),:);

    F1 = F1 + 2*(psi_i'*C'*Qy*C*phi_i);
    F2 = F2 - 2*(psi_i'*C'*Qy*Pi_nr_i);
    F3 = F3 - 2*(Pi_nu_i'*Qu);

    if i < N
        Pi_nu_2i = Pi_nu(((i+1)*nu)-(nu-1):(i+1)*(nu),:);
        H = H + 2*((psi_i'*C'*Qy*C*psi_i) + (Pi_nu_i'*Qu*Pi_nu_i) + (Pi_nu_2i - Pi_nu_i)'*Qu*(Pi_nu_2i - Pi_nu_i));

    else 
        H = H + 2*(psi_i'*C'*Qy*C*psi_i) + (Pi_nu_i'*Qu*Pi_nu_i);

    end

end

== matlab function QUAD_EULER_MPC_FTSMC3/Lineal MPC/MATLAB Function2 ==
  data: u input; y output
function y = fcn(u)

y = [u(1),u(2)]';

== matlab function QUAD_EULER_MPC_FTSMC3/Lineal MPC/MATLAB Function3 ==
  data: H input; y output; F input
function y = fcn(H,F)

y = (-H)\F;
